simulink model "Takeoff_Sim"  (R2023a)
settings: Solver=VariableStepAuto  StartTime=0.0  StopTime=35  RelTol=1e-3
values from neighbouring files (symbols this model uses):
  AoA = 5    [initialize.m]
  AR = 6.4897    [initialize.m]
  f = 6.271    [initialize.m]
  S = 174    [initialize.m]
  Weight = 2518    [initialize.m]
undefined symbols (not defined in the file or in its folder): Accelerometer, Accelerometerdeland, Earth, Gyroscope, Gyroscopedeland, Location, Locationdeland, WGS84
libraries: simulink_extras x10, aerolibtransform2 x4, simulink x4, aerolibatmos2 x2
(part 2 of 2)

== matlab function Takeoff_Sim/1D-INS (daytona)/total rotation ==
  data: Nx input; Nx_global output; Ny input; Nz input; roll input; Ny_global output; Nz_global output; pitch input; yaw input
function [Nx_global, Ny_global, Nz_global] = transform_attitude(Nx, Ny, Nz, roll, pitch, yaw)
% TRANSFORM_ATTITUDE - Rotates vectors Nx, Ny, Nz using roll, pitch, and yaw.
% INPUTS:
%   Nx, Ny, Nz       - Vector components in the local reference frame
%                     (Nx: forward, Ny: out the side, Nz: down)
%   roll             - Roll angle (rotation about Nx)
%   pitch            - Pitch angle (rotation about Ny)
%   yaw              - Yaw angle (rotation about Nz)
%   angle_in_degrees - Set to true if angles are in degrees, else false
% OUTPUTS:
%   Nx_global, Ny_global, Nz_global - Vector components in the global reference frame

    % Convert angles to radians if they are in degrees

    roll_rad  = deg2rad(roll);
    pitch_rad = deg2rad(pitch);
    yaw_rad   = deg2rad(yaw);


    % Rotation matrix for roll (about Nx)
    R_x = [1, 0,           0;
           0, cos(roll_rad), -sin(roll_rad);
           0, sin(roll_rad),  cos(roll_rad)];

    % Rotation matrix for pitch (about Ny)
    R_y = [cos(pitch_rad),  0, sin(pitch_rad);
           0,              1, 0;
          -sin(pitch_rad),  0, cos(pitch_rad)];

    % Rotation matrix for yaw (about Nz)
    R_z = [cos(yaw_rad), -sin(yaw_rad), 0;
           sin(yaw_rad),  cos(yaw_rad), 0;
           0,            0,           1];

    % Combined rotation matrix: yaw -> pitch -> roll
    R_combined = R_z * R_y * R_x;

    % Original vector in local frame
    N_local = [Nx; Ny; Nz];

    % Apply the combined rotation matrix
    N_global = R_combined * N_local;

    % Extract the components in the global reference frame
    Nx_global = N_global(1);
    Ny_global = N_global(2);
    Nz_global = N_global(3);
end

== matlab function Takeoff_Sim/1D-INS (Deland)/total rotation ==
  data: Nx input; Nx_global output; Ny input; Nz input; roll input; Ny_global output; Nz_global output; pitch input; yaw input
function [Nx_global, Ny_global, Nz_global] = transform_attitude(Nx, Ny, Nz, roll, pitch, yaw)
% TRANSFORM_ATTITUDE - Rotates vectors Nx, Ny, Nz using roll, pitch, and yaw.
% INPUTS:
%   Nx, Ny, Nz       - Vector components in the local reference frame
%                     (Nx: forward, Ny: out the side, Nz: down)
%   roll             - Roll angle (rotation about Nx)
%   pitch            - Pitch angle (rotation about Ny)
%   yaw              - Yaw angle (rotation about Nz)
%   angle_in_degrees - Set to true if angles are in degrees, else false
% OUTPUTS:
%   Nx_global, Ny_global, Nz_global - Vector components in the global reference frame

    % Convert angles to radians if they are in degrees

    roll_rad  = deg2rad(roll);
    pitch_rad = deg2rad(pitch);
    yaw_rad   = deg2rad(yaw);


    % Rotation matrix for roll (about Nx)
    R_x = [1, 0,           0;
           0, cos(roll_rad), -sin(roll_rad);
           0, sin(roll_rad),  cos(roll_rad)];

    % Rotation matrix for pitch (about Ny)
    R_y = [cos(pitch_rad),  0, sin(pitch_rad);
           0,              1, 0;
          -sin(pitch_rad),  0, cos(pitch_rad)];

    % Rotation matrix for yaw (about Nz)
    R_z = [cos(yaw_rad), -sin(yaw_rad), 0;
           sin(yaw_rad),  cos(yaw_rad), 0;
           0,            0,           1];

    % Combined rotation matrix: yaw -> pitch -> roll
    R_combined = R_z * R_y * R_x;

    % Original vector in local frame
    N_local = [Nx; Ny; Nz];

    % Apply the combined rotation matrix
    N_global = R_combined * N_local;

    % Extract the components in the global reference frame
    Nx_global = N_global(1);
    Ny_global = N_global(2);
    Nz_global = N_global(3);
end
